simulink model "practico_3"  (R2024b)
settings: Solver=FixedStepAuto  StartTime=0.0  StopTime=400  FixedStep=0.1  RelTol=1e-3
values from neighbouring files (symbols this model uses):
  F_in = 0.0035    [tp3_inicio.m]
  F_out_sin_k = a*sqrt(2*g)    [tp3_inicio.m]
  h_list = [0.2, 0.4, 0.6, 0.8]    [tp3_inicio.m]
  k_list = zeros(1, length(h_list))    [tp3_inicio.m]
  r_0 = 0.05    [tp3_inicio.m]
  theta = 60    [tp3_inicio.m]
undefined symbols (not defined in the file or in its folder): A, B, C, D
libraries: slpidlib x1
settings Model: Creator=trulscarlson  LastModifiedBy=trulscarlson
settings DebuggingCC: UnconnectedInputMsg=warning  UnconnectedOutputMsg=warning  UnconnectedLineMsg=warning
settings ModelReferenceCC: EnableRefExpFcnMdlSchedulingChecks=on
settings RTWCC: GPUComputeCapability=3.5  DLArmComputeVersion=19.05

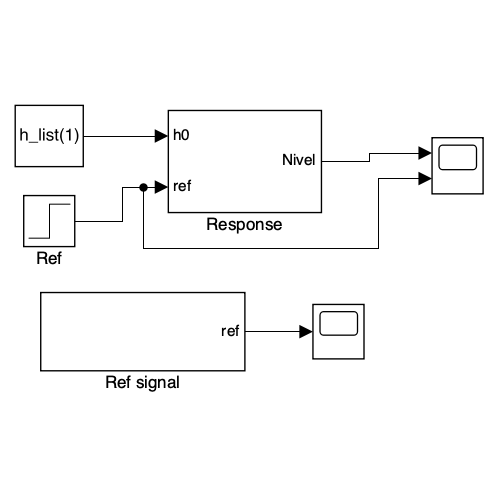
[thumbnail: Simulink's stored preview of the top-level diagram]
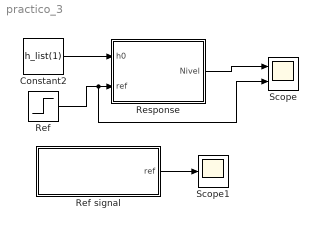
== system practico_3 ==
  Constant2 : Constant  Value=h_list(1)
  Ref : Step  Time=20  Before=h_list(1)  After=0.8  SampleTime=0
  Ref signal : Subsystem
  Response : Subsystem
  Scope : Scope  NumInputPorts=2
  Scope1 : Scope
  wires:
  Response/1(Nivel) -> Scope/1
  Constant2/1 -> Response/1(h0)
  Ref signal/1(ref) -> Scope1/1
  Ref/1 -> Scope/2, Response/2(ref)

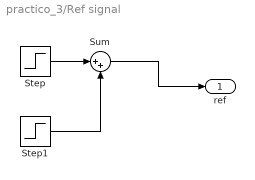
== system practico_3/Ref signal ==
  Step : Step  Time=40  Before=0.2  After=0.6  SampleTime=0
  Step1 : Step  Time=400  After=0.4  SampleTime=0
  Sum : Sum  Inputs=|++
  ref : Outport
  wires:
  Step1/1 -> Sum/2
  Step/1 -> Sum/1
  Sum/1 -> ref/1

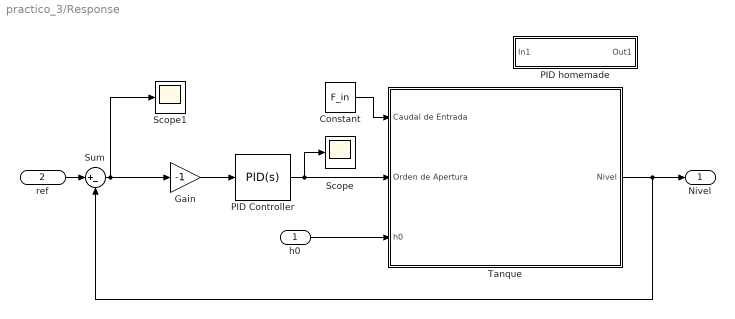
== system practico_3/Response ==
  h0 : Inport
  ref : Inport  Port=2
  Constant : Constant  Value=F_in
  Gain : Gain  Gain=-1
  PID Controller : slpidlib/PID Controller  Controller=PID  Form=Parallel  TimeDomain=Continuous-time  UseExternalTs=off  SampleTime=-1  IntegratorMethod=Forward Euler  FilterMethod=Forward Euler  ControllerParametersSource=internal  P=4  I=0.04  UseKiTs=off  D=50  UseExternalDerivativeSource=off  N=10  UseFilter=on  TunerSelectOption=Transfer Function Based (PID Tuner App)  InitialConditionSource=internal  InitialConditionForIntegrator=k_list(1)  InitialConditionForFilter=0  DifferentiatorICPrevScaledInput=0  ExternalReset=none  TrackingMode=off  Kt=1  LimitOutput=on  SatLimitsSource=internal  UpperSaturationLimit=1  LowerSaturationLimit=0  LinearizeAsGain=on  AntiWindupMode=clamping  Kb=1  LimitIntegrator=off  UpperIntegratorSaturationLimit=inf  LowerIntegratorSaturationLimit=-inf  POutMin=[]  POutMax=[]  IOutMin=[]  IOutMax=[]  DOutMin=[]  DOutMax=[]  NOutMin=[]  NOutMax=[]  SumOutMin=[]  SumOutMax=[]  SaturationOutMin=[]  SaturationOutMax=[]  PParamMin=[]  PParamMax=[]  IParamMin=[]  IParamMax=[]  DParamMin=[]  DParamMax=[]  NParamMin=[]  NParamMax=[]  KbParamMin=[]  KbParamMax=[]  KtParamMin=[]  KtParamMax=[]  KbOutMin=[]  KbOutMax=[]  KtOutMin=[]  KtOutMax=[]  IntegratorOutMin=[]  IntegratorOutMax=[]  FilterOutMin=[]  FilterOutMax=[]  SumI1OutMin=[]  SumI1OutMax=[]  SumI2OutMin=[]  SumI2OutMax=[]  SumI3OutMin=[]  SumI3OutMax=[]  SumI4OutMin=[]  SumI4OutMax=[]  SumDOutMin=[]  SumDOutMax=[]  DifferentiatorOutMin=[]  DifferentiatorOutMax=[]  FilterDiffOutCoefMin=[]  FilterDiffOutCoefMax=[]  ReciprocalOutMin=[]  ReciprocalOutMax=[]  SumDenOutMin=[]  SumDenOutMax=[]  SumNumOutMin=[]  SumNumOutMax=[]  DivideOutMin=[]  DivideOutMax=[]  UdiffTsProdOutMin=[]  UdiffTsProdOutMax=[]  NTsProdOutMin=[]  NTsProdOutMax=[]  UintegralTsProdOutMin=[]  UintegralTsProdOutMax=[]  UngainTsProdOutMin=[]  UngainTsProdOutMax=[]  ClampingZeroOutDataTypeStr=Inherit: Inherit via back propagation  ClampingZeroOutMin=[]  ClampingZeroOutMax=[]  FilterDenConstantOutDataTypeStr=Inherit: Inherit via back propagation  FilterDenConstantOutMin=[]  FilterDenConstantOutMax=[]  PCopyOutDataTypeStr=Inherit: Inherit via back propagation  PCopyOutMin=[]  PCopyOutMax=[]  NCopyOutDataTypeStr=Inherit: Inherit via back propagation  NCopyOutMin=[]  NCopyOutMax=[]  IntegratorContinuousStateAttributes=''  IntegratorStateMustResolveToSignalObject=off  IntegratorRTWStateStorageClass=Auto  FilterContinuousStateAttributes=''  FilterStateMustResolveToSignalObject=off  FilterRTWStateStorageClass=Auto  ParallelPVariant=InternalParameters  IdealPVariant=Disabled  IVariant=InternalParameters  DVariant=InternalParameters  IntegratorVariant=Continuous  SatVariant=Enabled  AWVariant=ContClampingParallel  PCopyVariant=Disabled  TRVariant=Disabled  FdbkBlocksVariant=Forward  IdealPFdbkVariant=Disabled  SatFdbkVariant=Disabled  DerivativeFilterVariant=ContFilter  NVariant=InternalParameters  NCopyVariant=Disabled  FilterICVariant=InternalICsFilter  IntegratorICVariant=InternalICs  ExternalResetVariant=Disabled  TRSumVariant=Passthrough  SumFdbkVariant=Disabled  SumVariant=Sum_PID  TsampFilterVariant=InternalTs  TsampNgainVariant=Passthrough  TsampIntegralVariant=Disabled_SignalSpec  ExternalSaturationOutDataTypeStr=Inherit: Same as second input  DerivativeSourceVariant=ErrorSignal  PreIntVariant=InternalPreInt
  PID homemade : Subsystem
  Scope : Scope
  Scope1 : Scope
  Sum : Sum  Inputs=|+-
  Tanque : Subsystem
  Nivel : Outport
  wires:
  h0/1 -> Tanque/3(h0)
  Constant/1 -> Tanque/1(Caudal de Entrada)
  Tanque/1(Nivel) -> Sum/2, Nivel/1
  ref/1 -> Sum/1
  Sum/1 -> Scope1/1, Gain/1
  PID Controller/1 -> Scope/1, Tanque/2(Orden de Apertura)
  Gain/1 -> PID Controller/1

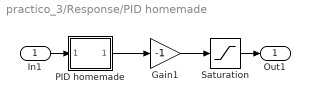
== system practico_3/Response/PID homemade ==
  In1 : Inport
  Gain1 : Gain  Gain=-1
  PID homemade : Subsystem
  Saturation : Saturate  UpperLimit=1  LowerLimit=0
  Out1 : Outport
  wires:
  In1/1 -> PID homemade/1(In1)
  Saturation/1 -> Out1/1
  Gain1/1 -> Saturation/1
  PID homemade/1(act) -> Gain1/1

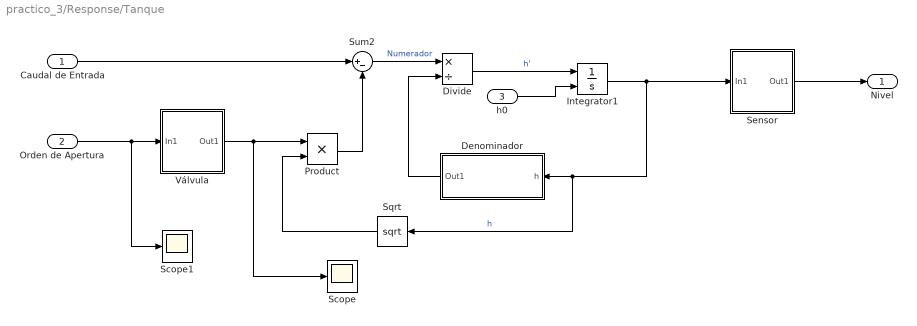
== system practico_3/Response/Tanque ==
  Caudal de Entrada : Inport
  Orden de Apertura : Inport  Port=2
  h0 : Inport  Port=3
  Denominador : Subsystem
  Divide : Product  Inputs=*/
  Integrator1 : Integrator  InitialConditionSource=external  InitialCondition=h_list(5)
  Product : Product
  Scope : Scope
  Scope1 : Scope
  Sensor : Subsystem
  Sqrt : Sqrt
  Sum2 : Sum  Inputs=|+-
  Válvula : Subsystem
  Nivel : Outport
  wires:
  Product/1 -> Sum2/2
  Divide/1 -> Integrator1/1  "h'"
  Denominador/1(Out1) -> Divide/2
  Integrator1/1 -> Sensor/1(In1), Sqrt/1, Denominador/1(h)  "h"
  Sum2/1 -> Divide/1  "Numerador"
  Sqrt/1 -> Product/2
  Caudal de Entrada/1 -> Sum2/1
  Orden de Apertura/1 -> Válvula/1(In1), Scope1/1
  Válvula/1(Out1) -> Product/1, Scope/1
  h0/1 -> Integrator1/2
  Sensor/1(Out1) -> Nivel/1

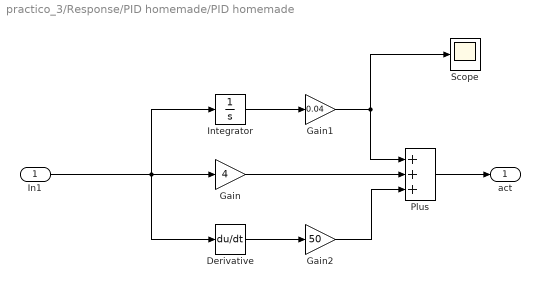
== system practico_3/Response/PID homemade/PID homemade ==
  In1 : Inport
  Derivative : Derivative
  Gain : Gain  Gain=4
  Gain1 : Gain  Gain=0.04
  Gain2 : Gain  Gain=50
  Integrator : Integrator
  Plus : Sum  Inputs=+++
  Scope : Scope
  act : Outport
  wires:
  In1/1 -> Derivative/1, Integrator/1, Gain/1
  Integrator/1 -> Gain1/1
  Gain1/1 -> Scope/1, Plus/1
  Plus/1 -> act/1
  Derivative/1 -> Gain2/1
  Gain/1 -> Plus/2
  Gain2/1 -> Plus/3

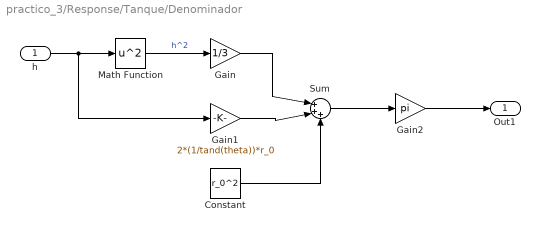
== system practico_3/Response/Tanque/Denominador ==
  h : Inport
  Constant : Constant  Value=r_0^2
  Gain : Gain  Gain=1/3
  Gain1 : Gain  Gain=2*(1/tand(theta))*r_0
  Gain2 : Gain  Gain=pi
  Math Function : Math  Operator=square
  Sum : Sum  Inputs=|+++
  Out1 : Outport
  wires:
  h/1 -> Gain1/1, Math Function/1
  Math Function/1 -> Gain/1  "h^2"
  Gain/1 -> Sum/1
  Gain1/1 -> Sum/2
  Constant/1 -> Sum/3
  Sum/1 -> Gain2/1
  Gain2/1 -> Out1/1

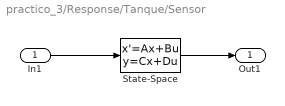
== system practico_3/Response/Tanque/Sensor ==
  In1 : Inport
  State-Space : StateSpace  A=A  B=B  C=C  D=D  InitialCondition=h_list(1)*10
  Out1 : Outport
  wires:
  In1/1 -> State-Space/1
  State-Space/1 -> Out1/1

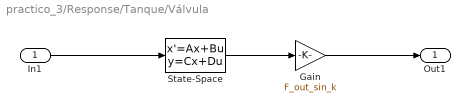
== system practico_3/Response/Tanque/Válvula ==
  In1 : Inport
  Gain : Gain  Gain=F_out_sin_k
  State-Space : StateSpace  A=A  B=B  C=C  D=D  InitialCondition=k_list(1)*10
  Out1 : Outport
  wires:
  State-Space/1 -> Gain/1
  Gain/1 -> Out1/1
  In1/1 -> State-Space/1
